simulink model "Modelo_1gdl_PID_R2025a"  (R2025a)
settings: Solver=FixedStepDiscrete  StartTime=0.0  StopTime=pid1_t_stop  FixedStep=pid_dt  RelTol=1e-3  EnableMultiTasking=on
InitFcn:
  | run('C:\00_Research_\Neuromorphic_Embodied_AI\02_Coaxial_TriRotor_Nengo\baseline_victor\PID_R2025a_models\params\victor_pid_params.m')
undefined symbols (not defined in the file): pid1_int0, pid1_param_vec, pid1_x0, pid_dt
settings Model: ExtModeTrigDuration=10000  Creator=gandhico  LastModifiedBy=gandhico
settings SolverCC: AlgebraicLoopSolver=TrustRegion  PositivePriorityOrder=on
settings DataIOCC: ReturnWorkspaceOutputs=off
settings DebuggingCC: UnconnectedInputMsg=warning  UnconnectedOutputMsg=warning  UnconnectedLineMsg=warning  ArithmeticOperatorsInVariantConditions=warning
settings ModelReferenceCC: EnableRefExpFcnMdlSchedulingChecks=on
settings SFSimCC: SimUseLocalCustomCode=off  CustomCodeUndefinedFunction=UseInterfaceOnly
settings RTWCC: SystemTargetFile=quarc_win64.tlc  TemplateMakefile=quarc_default_tmf  RTWUseLocalCustomCode=off  Toolchain=QUARC win64 | nmake (64-bit Windows)  BuildConfiguration=Faster Runs  GPUComputeCapability=3.5  Description=QUARC Win64 Target Using Toolchain
settings CodeAppCC: StateflowObjectComments=on
settings STFCustomTargetCC: SystemTargetFile=quarc_win64.tlc  TargetLangStandard=C99 (ISO)  MultiwordLength=2048.0  DynamicStringBufferSize=256.0  ConcurrentExecutionCompliant=on  UseToolchainInfoCompliant=on
settings GRTTargetCC: ExtMode=on  ExtModeMexFile=quarc_comm  ParMdlRefBuildCompliant=off  CompOptLevelCompliant=off  CombineOutputUpdateFcns=off  MatFileLogging=off  CPPClassGenCompliant=off  GRTInterface=on
settings ConfigComp: CovMetricSettings=dswe

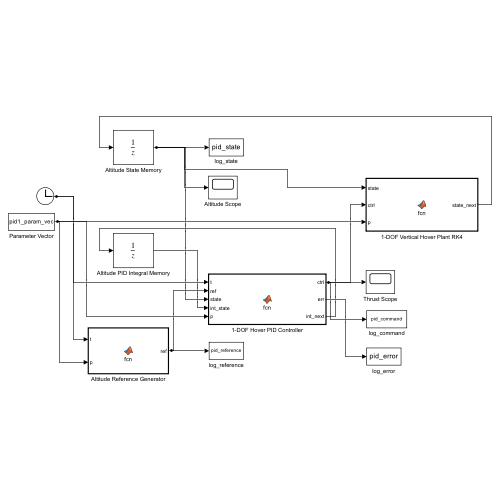
[thumbnail: Simulink's stored preview of the top-level diagram]
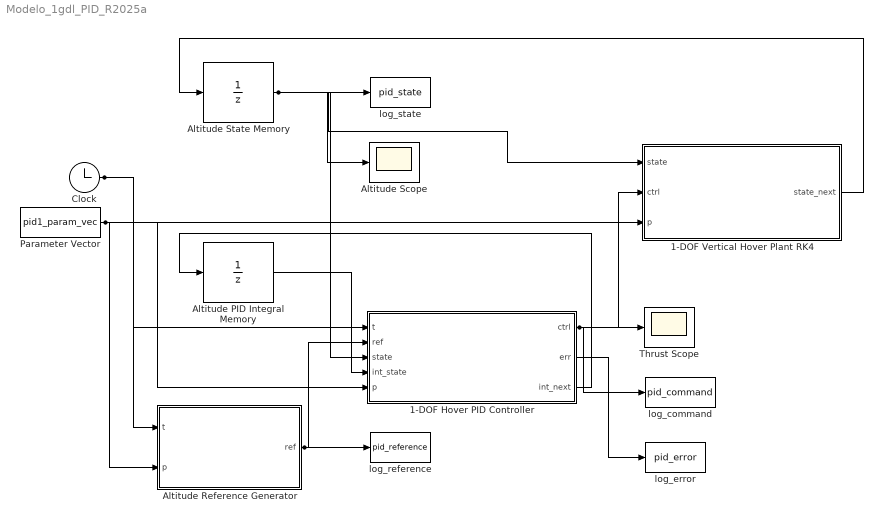
== system Modelo_1gdl_PID_R2025a ==
  1-DOF Hover PID Controller : MATLAB Function  TreatAsAtomicUnit=on
  1-DOF Vertical Hover Plant RK4 : MATLAB Function  TreatAsAtomicUnit=on
  Altitude PID Integral Memory : UnitDelay  InitialCondition=pid1_int0  SampleTime=pid_dt  HasFrameUpgradeWarning=on
  Altitude Reference Generator : MATLAB Function  TreatAsAtomicUnit=on
  Altitude Scope : Scope
  Altitude State Memory : UnitDelay  InitialCondition=pid1_x0  SampleTime=pid_dt  HasFrameUpgradeWarning=on
  Clock : Clock
  Parameter Vector : Constant  Value=pid1_param_vec
  Thrust Scope : Scope
  log_command : ToWorkspace  VariableName=pid_command  SaveFormat=Structure With Time  SampleTime=-1
  log_error : ToWorkspace  VariableName=pid_error  SaveFormat=Structure With Time  SampleTime=-1
  log_reference : ToWorkspace  VariableName=pid_reference  SaveFormat=Structure With Time  SampleTime=-1
  log_state : ToWorkspace  VariableName=pid_state  SaveFormat=Structure With Time  SampleTime=-1
  wires:
  1-DOF Hover PID Controller/2(err) -> log_error/1
  Clock/1 -> 1-DOF Hover PID Controller/1(t), Altitude Reference Generator/1(t)
  Altitude PID Integral Memory/1 -> 1-DOF Hover PID Controller/4(int_state)
  Parameter Vector/1 -> 1-DOF Vertical Hover Plant RK4/3(p), 1-DOF Hover PID Controller/5(p), Altitude Reference Generator/2(p)
  Altitude State Memory/1 -> 1-DOF Vertical Hover Plant RK4/1(state), 1-DOF Hover PID Controller/3(state), log_state/1, Altitude Scope/1
  Altitude Reference Generator/1(ref) -> 1-DOF Hover PID Controller/2(ref), log_reference/1
  1-DOF Hover PID Controller/3(int_next) -> Altitude PID Integral Memory/1
  1-DOF Hover PID Controller/1(ctrl) -> 1-DOF Vertical Hover Plant RK4/2(ctrl), Thrust Scope/1, log_command/1
  1-DOF Vertical Hover Plant RK4/1(state_next) -> Altitude State Memory/1

== matlab function Modelo_1gdl_PID_R2025a/1-DOF Hover PID Controller ==
  data: t input size=[1 1]; ctrl output size=[6 1]; ref input size=[2 1]; state input size=[2 1]; int_state input size=[1 1]; p input size=[14 1]; err output size=[3 1]; int_next output size=[1 1]
function [ctrl, err, int_next] = fcn(t, ref, state, int_state, p)
%#codegen
pid_dt = p(1);
m = p(2);
g = p(3);
Kp = p(9);
Ki = p(10);
Kd = p(11);
int_limit = p(12);
T_min = p(13);
T_max = p(14);

z = state(1);
dz = state(2);
e = ref(1) - z;
edot = ref(2) - dz;
e_int = min(max(int_state(1) + pid_dt*e, -int_limit), int_limit);

feedforward = m*g;
T_unsat = Kp*e + Ki*e_int + Kd*edot + feedforward;
T = min(max(T_unsat, T_min), T_max);

ctrl = [T; T_unsat; feedforward; e; e_int; edot];
err = [e; e_int; edot];
int_next = e_int;
end

== matlab function Modelo_1gdl_PID_R2025a/Altitude Reference Generator ==
  data: t input size=[1 1]; ref output size=[2 1]; p input size=[14 1]
function ref = fcn(t, p)
%#codegen
k = p(6);
amp = p(7);
center = p(8);
q = exp(-k*(t - center));
den = 1.0 + q;
z_ref = amp/den;
dz_ref = amp*k*q/(den*den);
ref = [z_ref; dz_ref];
end

== matlab function Modelo_1gdl_PID_R2025a/1-DOF Vertical Hover Plant RK4 ==
  data: state input size=[2 1]; state_next output size=[2 1]; ctrl input size=[6 1]; p input size=[14 1]
function state_next = fcn(state, ctrl, p)
%#codegen
h = p(1);
T = ctrl(1);
k1 = dyn_1gdl(state, T, p);
k2 = dyn_1gdl(state + 0.5*h*k1, T, p);
k3 = dyn_1gdl(state + 0.5*h*k2, T, p);
k4 = dyn_1gdl(state + h*k3, T, p);
state_next = state + (h/6.0)*(k1 + 2.0*k2 + 2.0*k3 + k4);
end

function dx = dyn_1gdl(x, T, p)
m = p(2);
g = p(3);
theta = p(4);
phi = p(5);
z_dot = x(2);
z_ddot = (T/m)*cos(theta)*cos(phi) - g;
dx = [z_dot; z_ddot];
end
